simulink model "encoder"  (R2018b)
settings: Solver=FixedStepDiscrete  StartTime=0.0  StopTime=10.0  RelTol=1e-3
libraries: hdlsllib x12
settings Model: Creator=jayakumarav  LastModifiedBy=hiterd
settings DebuggingCC: LibraryContextMissingDiagnostic=none
settings SFSimCC: SimUseLocalCustomCode=off
settings RTWCC: RTWUseLocalCustomCode=off

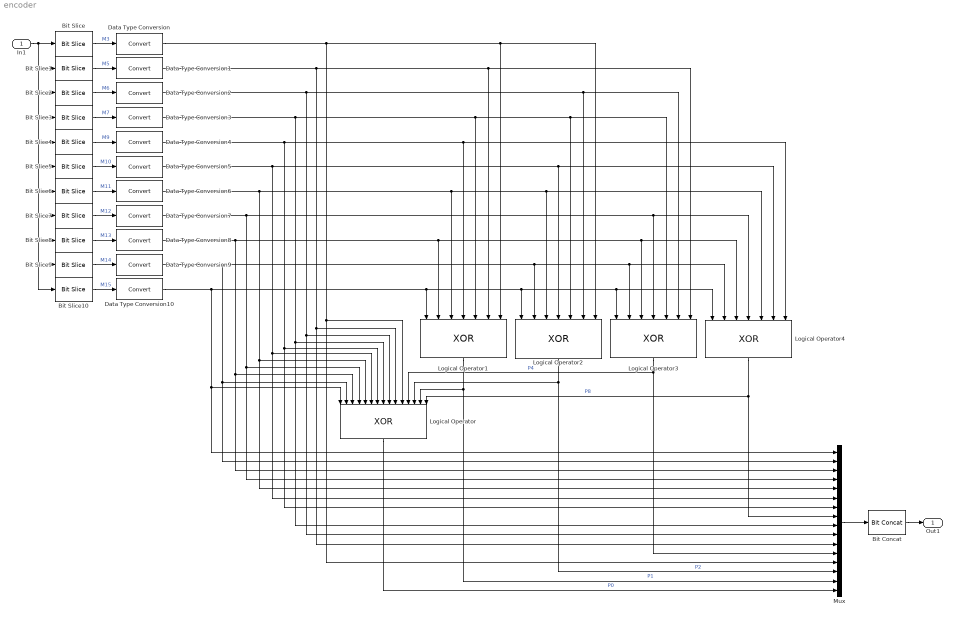
== system encoder ==
  In1 : Inport  OutDataTypeStr=int32  PortDimensions=1
  Bit Concat : hdlsllib/Logic and Bit Operations/Bit Concat  numInputs=1
      settings: SourceProductName=HDL Coder  SourceProductBaseCode=HD
  Bit Slice : hdlsllib/Logic and Bit Operations/Bit Slice  lidx=0  ridx=0
  Bit Slice1 : hdlsllib/Logic and Bit Operations/Bit Slice  lidx=1  ridx=1
  Bit Slice10 : hdlsllib/Logic and Bit Operations/Bit Slice  lidx=10  ridx=10
  Bit Slice2 : hdlsllib/Logic and Bit Operations/Bit Slice  lidx=2  ridx=2
  Bit Slice3 : hdlsllib/Logic and Bit Operations/Bit Slice  lidx=3  ridx=3
  Bit Slice4 : hdlsllib/Logic and Bit Operations/Bit Slice  lidx=4  ridx=4
  Bit Slice5 : hdlsllib/Logic and Bit Operations/Bit Slice  lidx=5  ridx=5
  Bit Slice6 : hdlsllib/Logic and Bit Operations/Bit Slice  lidx=6  ridx=6
  Bit Slice7 : hdlsllib/Logic and Bit Operations/Bit Slice  lidx=7  ridx=7
  Bit Slice8 : hdlsllib/Logic and Bit Operations/Bit Slice  lidx=8  ridx=8
  Bit Slice9 : hdlsllib/Logic and Bit Operations/Bit Slice  lidx=9  ridx=9
  Data Type Conversion{,1..10} (11 alike) : DataTypeConversion
  Logical Operator : Logic  Operator=XOR  Inputs=15  IconShape=distinctive  AllPortsSameDT=off  OutDataTypeStr=boolean
  Logical Operator{1..4} (4 alike) : Logic  Operator=XOR  Inputs=7  IconShape=distinctive  AllPortsSameDT=off  OutDataTypeStr=boolean
  Mux : Mux  Inputs=16
  Out1 : Outport
  wires:
  Logical Operator/1 -> Mux/16  "P0"
  Logical Operator1/1 -> Mux/15, Logical Operator/14  "P1"
  Logical Operator2/1 -> Mux/14, Logical Operator/13  "P2"
  Logical Operator3/1 -> Mux/12, Logical Operator/12  "P4"
  Bit Slice1/1 -> Data Type Conversion1/1  "M5"
  Bit Slice2/1 -> Data Type Conversion2/1  "M6"
  Bit Slice3/1 -> Data Type Conversion3/1  "M7"
  Bit Slice4/1 -> Data Type Conversion4/1  "M9"
  Bit Slice5/1 -> Data Type Conversion5/1  "M10"
  Bit Slice6/1 -> Data Type Conversion6/1  "M11"
  Bit Slice7/1 -> Data Type Conversion7/1  "M12"
  Bit Slice9/1 -> Data Type Conversion9/1  "M14"
  Bit Slice10/1 -> Data Type Conversion10/1  "M15"
  Logical Operator4/1 -> Mux/8, Logical Operator/15  "P8"
  Bit Slice/1 -> Data Type Conversion/1  "M3"
  In1/1 -> Bit Slice3/1, Bit Slice4/1, Bit Slice5/1, Bit Slice6/1, Bit Slice7/1, Bit Slice8/1, Bit Slice9/1, Bit Slice10/1, Bit Slice2/1, Bit Slice1/1, Bit Slice/1
  Bit Slice8/1 -> Data Type Conversion8/1  "M13"
  Data Type Conversion/1 -> Logical Operator2/7, Logical Operator1/7, Mux/13, Logical Operator/11
  Data Type Conversion1/1 -> Logical Operator3/7, Logical Operator1/6, Mux/11, Logical Operator/10
  Data Type Conversion2/1 -> Logical Operator3/6, Logical Operator2/6, Mux/10, Logical Operator/9
  Data Type Conversion3/1 -> Logical Operator3/5, Logical Operator2/5, Logical Operator1/5, Mux/9, Logical Operator/8
  Data Type Conversion4/1 -> Logical Operator4/7, Logical Operator1/4, Mux/7, Logical Operator/7
  Data Type Conversion5/1 -> Logical Operator4/6, Logical Operator2/4, Mux/6, Logical Operator/6
  Data Type Conversion6/1 -> Logical Operator4/5, Logical Operator2/3, Logical Operator1/3, Mux/5, Logical Operator/5
  Data Type Conversion7/1 -> Logical Operator4/4, Logical Operator3/4, Mux/4, Logical Operator/4
  Data Type Conversion8/1 -> Logical Operator4/3, Logical Operator3/3, Logical Operator1/2, Mux/3, Logical Operator/3
  Data Type Conversion9/1 -> Logical Operator4/2, Logical Operator3/2, Logical Operator2/2, Mux/2, Logical Operator/2
  Data Type Conversion10/1 -> Logical Operator4/1, Logical Operator3/1, Logical Operator2/1, Logical Operator1/1, Logical Operator/1, Mux/1
  Mux/1 -> Bit Concat/1
  Bit Concat/1 -> Out1/1
